simulink model "Test_16B_Memory_Block"  (Simulink 8.1)
settings: Solver=ode45  StartTime=0.0  StopTime=10.0  RelTol=1e-3
libraries: Computer_Library x1
settings Model: Creator=N  LastModifiedBy=uzivatel
settings DataIOCC: LimitDataPoints=off  SignalLoggingSaveFormat=Dataset
settings OptimizationCC: ExpressionDepthLimit=128
settings DebuggingCC: UnderspecifiedInitializationDetection=Simplified  MergeDetectMultiDrivingBlocksExec=error  SolverPrmCheckMsg=none  FcnCallInpInsideContextMsg=EnableAllAsError  FrameProcessingCompatibilityMsg=error  StateNameClashWarn=none
settings HardwareCC: ProdBitPerPointer=64  ProdLargestAtomicFloat=Float  ProdIntDivRoundTo=Zero  ProdEndianess=LittleEndian  ProdHWDeviceType=Intel->x86-64 (Windows64)
settings ModelReferenceCC: PropagateSignalLabelsOutOfModel=on
settings GRTTargetCC: CodeReplacementLibrary=None  CombineOutputUpdateFcns=on  CPPClassGenCompliant=on  GRTInterface=off

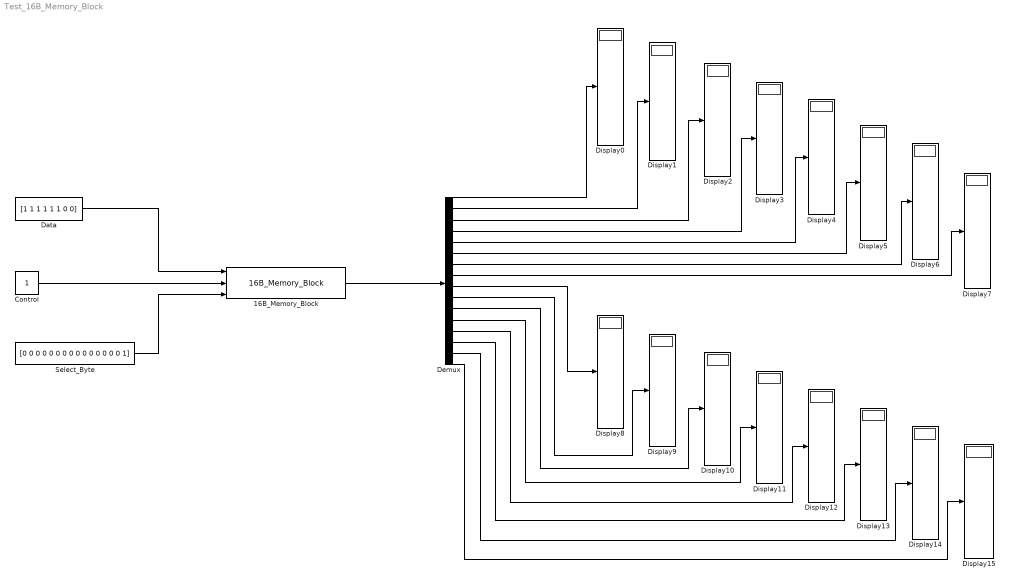
== system Test_16B_Memory_Block ==
  16B_Memory_Block : Computer_Library/16B_Memory_Block
  Control : Constant
  Data : Constant  Value=[1 1 1 1 1 1 0 0]  OutDataTypeStr=boolean
  Demux : Demux  Outputs=16
  Display{0..15} (16 alike) : Display
  Select_Byte : Constant  Value=[0 0 0 0 0 0 0 0 0 0 0 0 0 0 0 1]  OutDataTypeStr=boolean
  wires:
  16B_Memory_Block/1 -> Demux/1
  Demux/1 -> Display0/1
  Demux/2 -> Display1/1
  Demux/3 -> Display2/1
  Demux/4 -> Display3/1
  Demux/5 -> Display4/1
  Demux/6 -> Display5/1
  Demux/7 -> Display6/1
  Demux/8 -> Display7/1
  Demux/9 -> Display8/1
  Demux/10 -> Display9/1
  Demux/11 -> Display10/1
  Demux/12 -> Display11/1
  Demux/13 -> Display12/1
  Demux/14 -> Display13/1
  Demux/15 -> Display14/1
  Demux/16 -> Display15/1
  Data/1 -> 16B_Memory_Block/1
  Control/1 -> 16B_Memory_Block/2
  Select_Byte/1 -> 16B_Memory_Block/3
